simulink model "T7_bloques"  (R2025a)
settings: Solver=VariableStepAuto  StartTime=0.0  StopTime=10.0  RelTol=1e-3
InitFcn:
  | Ra = 2;
  | Kt = 0.01;
  | b = 0.0012;
  | La = 0.023;
  | Ke = 0.01;
  | Jm = 0.001;
settings Model: Creator=carlo  LastModifiedBy=carlo

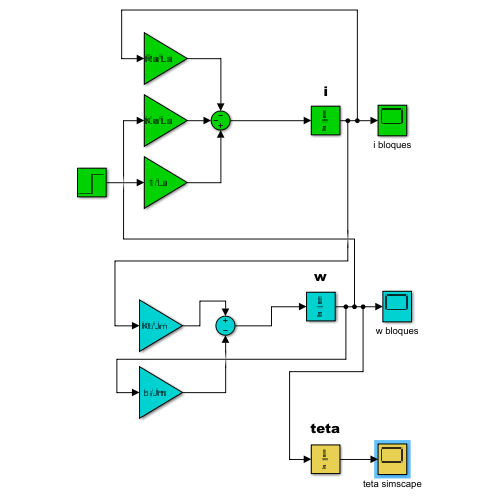
[thumbnail: Simulink's stored preview of the top-level diagram]
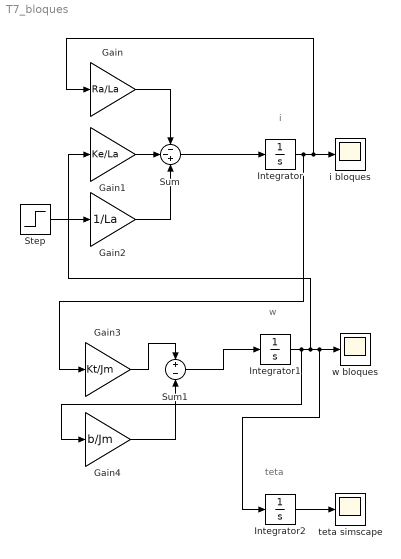
== system T7_bloques ==
  note: i
  note: w
  note: teta
  Gain : Gain  Gain=Ra/La
  Gain1 : Gain  Gain=Ke/La
  Gain2 : Gain  Gain=1/La
  Gain3 : Gain  Gain=Kt/Jm
  Gain4 : Gain  Gain=b/Jm
  Integrator : Integrator
  Integrator1 : Integrator
  Integrator2 : Integrator
  Step : Step  Before=1  SampleTime=0
  Sum : Sum  Inputs=--+
  Sum1 : Sum  Inputs=+-
  i bloques : Scope
      settings: ActiveDisplayYMinimum=-0.062270632804103228  ActiveDisplayYMaximum=0.56043569523692915
  teta simscape : Scope
      settings: ActiveDisplayYMinimum=-4.5944814863865542  ActiveDisplayYMaximum=41.350333377479  DataLoggingVariableName=ScopeData2
  w bloques : Scope
      settings: ActiveDisplayYMinimum=-0.5000051462553976  ActiveDisplayYMaximum=4.5000463162985795
  wires:
  Sum/1 -> Integrator/1
  Gain/1 -> Sum/1
  Integrator/1 -> Gain3/1, Gain/1, i bloques/1
  Integrator1/1 -> Gain1/1, Integrator2/1, w bloques/1, Gain4/1
  Integrator2/1 -> teta simscape/1
  Gain1/1 -> Sum/2
  Gain2/1 -> Sum/3
  Step/1 -> Gain2/1
  Gain3/1 -> Sum1/1
  Gain4/1 -> Sum1/2
  Sum1/1 -> Integrator1/1
